simulink model "kapitsa_pendulum"  (R2021b)
settings: Solver=VariableStepAuto  StartTime=0.0  StopTime=5  MaxStep=0.05  RelTol=1e-3
undefined symbols (not defined in the file): amplitude, decrement, frequency, lenght, start_angle
libraries: simulink_extras x1
settings Model: Creator=USER  LastModifiedBy=USER
settings DataIOCC: ReturnWorkspaceOutputs=off

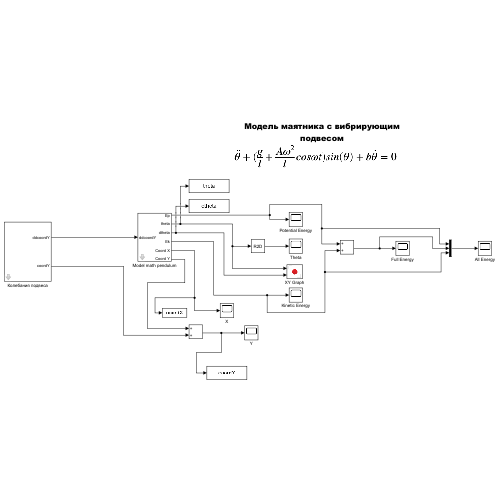
[thumbnail: Simulink's stored preview of the top-level diagram]
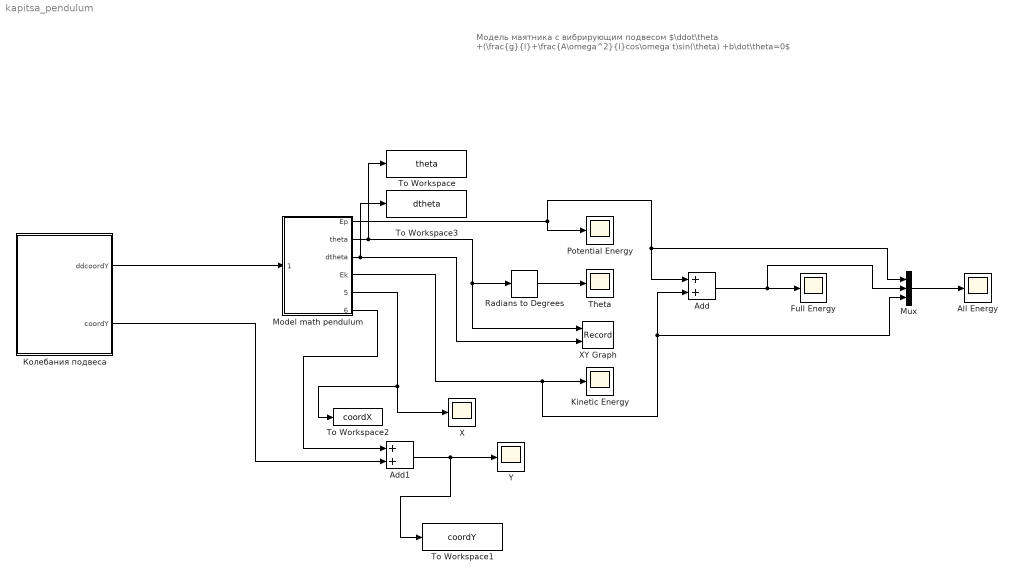
== system kapitsa_pendulum ==
  note: Модель маятника с вибрирующим подвесом
      | $\ddot\theta +(\frac{g}{l}+\frac{A\omega^2}{l}cos\omega t)sin(\theta) +b\dot\theta=0$
  Add : Sum
  Add1 : Sum
  All Energy : Scope
  Full Energy : Scope
  Kinetic Energy : Scope
  Model math pendulum : Subsystem  mask{m=1, l=lenght, g=9.8, start_angle_deg=start_angle, b=decrement}
      mask prompts: m "Mass"; l "Length"; g "Acceleration free downfall"; start_angle_deg "Start angle"; b "Dissipative member"
      mask init:
      | I = m * l^2
  Mux : Mux  Inputs=3
  Potential Energy : Scope
  Radians to Degrees : simulink_extras/Transformations/Radians to Degrees
  Theta : Scope
  To Workspace : ToWorkspace  VariableName=theta  SampleTime=-1
      settings: Save2DSignal=2-D array (concatenate along first dimension)
  To Workspace1 : ToWorkspace  VariableName=coordY  SampleTime=-1
      settings: Save2DSignal=2-D array (concatenate along first dimension)
  To Workspace2 : ToWorkspace  VariableName=coordX  SampleTime=-1
      settings: Save2DSignal=2-D array (concatenate along first dimension)
  To Workspace3 : ToWorkspace  VariableName=dtheta  SampleTime=-1
      settings: Save2DSignal=2-D array (concatenate along first dimension)
  X : Scope
  XY Graph : Record  FileSettingsInternal="{\"entries\":[{\"content\":{\"excelSettings\":{\"content\":{},\"type\":\"Streamout.ExcelSettings\"}},\"type\":\"Streamout.FileSettingStorage\",\"uuid\":\"75ce60ae-1aaa-4546-8ea2-1419d0a5cab1\"}],\"packageUris\":[\"http://schema.mathworks.com/mf0/streamout_blocks/R2020a\"],\"version\":\"1.0\"}"  Layout=[1 1]  SignalsInternal="{\"entries\":[{\"content\":{\"signals\":[{\"content\":{\"blockPath\":[\"kapitsa_pendulum/XY Graph\"],\"channel\":[],\"dimensions\":[1],\"domain\":\"kapitsa_pendulum/XY Graph\",\"lineColor\":\"#a2142f\",\"plots\":[1],\"port\":1,\"sid\":[\"\"],\"signalID\":1275,\"signalName\":\"Model math pendulum:2\"},\"type\":\"RecordBlkView.Signal\",\"uuid\":\"31c1e4ce-d13d-4d3d-a56a-d89802a88d0b\"},{\"content\":{\"blockPath\":[\"kapitsa_pendulum/XY Graph\"],\"channel\":[],\"dimensions\":[1],\"domain\":\"kapitsa_pendulum/XY Graph\",\"lineColor\":\"#139fff\",\"plots\":[1],\"port\":2,\"sid\":[\"\"],\"signalID\":1279,\"signalName\":\"Model math pendulum:3\"},\"type\":\"RecordBlkView.Signal\",\"uuid\":\"8315b68a-bbb4-4935-805b-d24630a1185a\"}]},\"type\":\"RecordBlkView.InputSignals\",\"uuid\":\"e2399d69-aa14-42c6-a3e5-5ebebae03b7e\"}],\"packageUris\":[\"http://schema.mathworks.com/mf0/streamout_blocks/R2020a\"],\"version\":\"1.0\"}"  VisualizationBindings="{\"xyplotplugin\":{\"info\":[{\"series\":[{\"bindingParametersList\":[{\"parameter\":\"X-Axis\",\"signalID\":1275,\"signalName\":\"Model math pendulum:2\"},{\"parameter\":\"Y-Axis\",\"signalID\":1279,\"signalName\":\"Model math pendulum:3\"}],\"seriesID\":22332}],\"subplotID\":1}]}}"  CompatibilityTag=XY
  Y : Scope
  Колебания подвеса : Subsystem  mask{w=frequency, A=amplitude}
      mask prompts: A "Amplitude"
  wires:
  Model math pendulum/5(Coord X) -> To Workspace2/1, X/1
  Add/1 -> Mux/2, Full Energy/1
  Model math pendulum/1(Ep) -> Potential Energy/1, Mux/1, Add/1
  Model math pendulum/2(theta) -> XY Graph/1, Radians to Degrees/1, To Workspace/1
  Model math pendulum/4(Ek) -> Mux/3, Add/2, Kinetic Energy/1
  Model math pendulum/3(dtheta) -> XY Graph/2, To Workspace3/1
  Mux/1 -> All Energy/1
  Radians to Degrees/1 -> Theta/1
  Колебания подвеса/2(coordY) -> Add1/2
  Колебания подвеса/1(ddcoordY) -> Model math pendulum/1(ddcoordY)
  Model math pendulum/6(Coord Y) -> Add1/1
  Add1/1 -> To Workspace1/1, Y/1

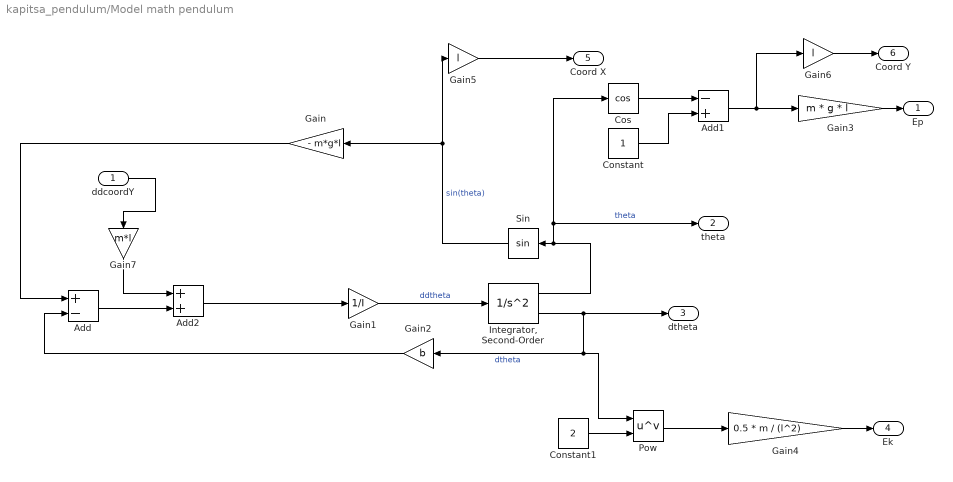
== system kapitsa_pendulum/Model math pendulum ==
  ddcoordY : Inport
  Add : Sum  Inputs=+-
  Add1 : Sum  Inputs=-+
  Add2 : Sum
  Constant : Constant
  Constant1 : Constant  Value=2
  Cos : Trigonometry  Operator=cos
  Gain : Gain  Gain=- m*g*l
  Gain1 : Gain  Gain=1/I
  Gain2 : Gain  Gain=b
  Gain3 : Gain  Gain=m * g * l
  Gain4 : Gain  Gain=0.5 * m / (l^2)
  Gain5 : Gain  Gain=l
  Gain6 : Gain  Gain=l
  Gain7 : Gain  Gain=m*l
  "Integrator, Second-Order" : SecondOrderIntegrator  ICX=deg2rad(start_angle_deg)
  Pow : Math  Operator=pow  SignedPower=on  RndMeth=Zero  SaturateOnIntegerOverflow=on
  Sin : Trigonometry
  Ep : Outport
  theta : Outport  Port=2
  dtheta : Outport  Port=3
  Ek : Outport  Port=4
  Coord X : Outport  Port=5
  Coord Y : Outport  Port=6
  wires:
  Gain1/1 -> "Integrator, Second-Order"/1  "ddtheta"
  "Integrator, Second-Order"/2 -> Pow/1, Gain2/1, dtheta/1  "dtheta"
  Sin/1 -> Gain5/1, Gain/1  "sin(theta)"
  "Integrator, Second-Order"/1 -> Cos/1, theta/1, Sin/1  "theta"
  Gain/1 -> Add/1
  Gain2/1 -> Add/2
  Add/1 -> Add2/2
  Gain3/1 -> Ep/1
  Add1/1 -> Gain6/1, Gain3/1
  Constant/1 -> Add1/2
  Pow/1 -> Gain4/1
  Gain4/1 -> Ek/1
  Constant1/1 -> Pow/2
  Gain5/1 -> Coord X/1
  Gain6/1 -> Coord Y/1
  Cos/1 -> Add1/1
  ddcoordY/1 -> Gain7/1
  Gain7/1 -> Add2/1
  Add2/1 -> Gain1/1

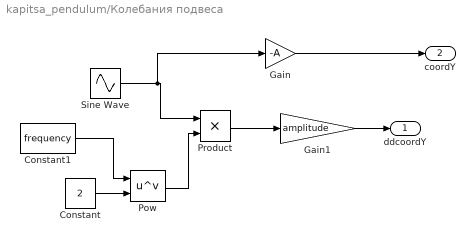
== system kapitsa_pendulum/Колебания подвеса ==
  Constant : Constant  Value=2
  Constant1 : Constant  Value=frequency
  Gain : Gain  Gain=-A
  Gain1 : Gain  Gain=amplitude
  Pow : Math  Operator=pow  SignedPower=on  RndMeth=Zero  SaturateOnIntegerOverflow=on
  Product : Product
  Sine Wave : Sin  Frequency=w*6.28  Phase=3.14/2  SampleTime=0
  ddcoordY : Outport
  coordY : Outport  Port=2
  wires:
  Pow/1 -> Product/2
  Constant/1 -> Pow/2
  Constant1/1 -> Pow/1
  Sine Wave/1 -> Gain/1, Product/1
  Product/1 -> Gain1/1
  Gain1/1 -> ddcoordY/1
  Gain/1 -> coordY/1
